simulink model "dbl_pendulum_total"  (R2021b)
settings: Solver=VariableStepAuto  StartTime=0.0  StopTime=10.0  RelTol=1e-3
values from neighbouring files (symbols this model uses):
  h = 0.001    [PID.m]    (also in blackbox_inpsig.m = fugiboard('Open', 'pendulum1'); blackbox_test.m = fugiboard('Open', 'pendulum1'); dbl_pend_blackbox_v1.m = fugiboard('Open', 'pendulum1'); dbl_pend_param_id_final.m)
libraries: eeLuenbergerObserver x1
settings Model: Creator=MICHAEL-LT  LastModifiedBy=mfuser
settings DataIOCC: ReturnWorkspaceOutputs=off

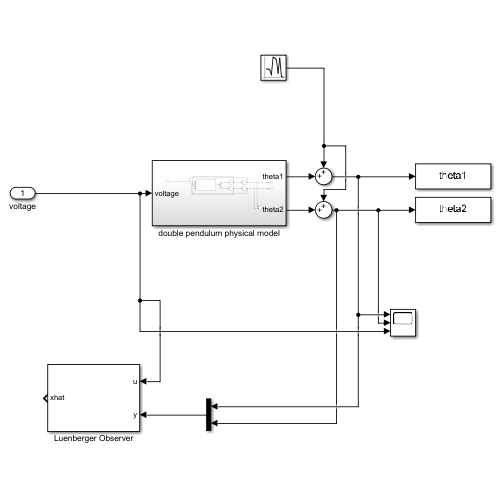
[thumbnail: Simulink's stored preview of the top-level diagram]
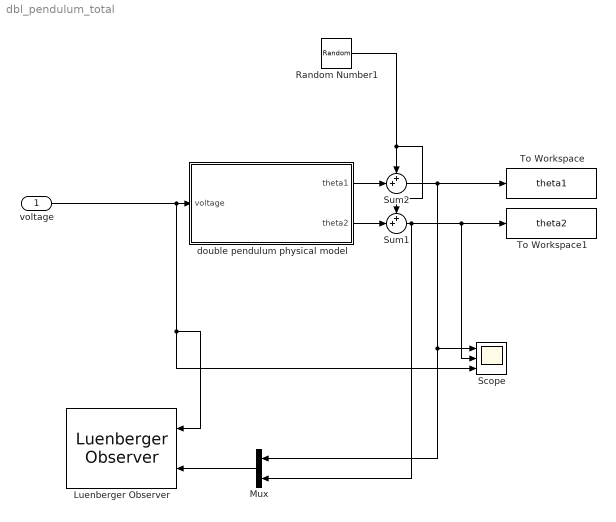
== system dbl_pendulum_total ==
  voltage : Inport
  Luenberger Observer : eeLuenbergerObserver/Luenberger Observer  StateSpaceType=Discrete-time  Ad=A_discr  Bd=B_discr  Cd=C_discr  Dd=D_discr  A=1  B=1  C=1  D=1  ObserverDesign=Observer gain  Ld=1  DesiredEigenvalues=0  x0=[0;0;0;0]  Tsd=0.1  Ts=h
      settings: SourceProductBaseCode=PS
  Mux : Mux  Inputs=2
  Random Number1 : RandomNumber  Variance=1e-5  SampleTime=h
  Scope : Scope  NumInputPorts=3
  Sum1 : Sum  Inputs=++|  SaturateOnIntegerOverflow=on
  Sum2 : Sum  Inputs=++|  SaturateOnIntegerOverflow=on
  To Workspace : ToWorkspace  VariableName=theta1  SampleTime=h
  To Workspace1 : ToWorkspace  VariableName=theta2  SampleTime=h
  double pendulum physical model : Subsystem
  wires:
  voltage/1 -> Scope/3, Luenberger Observer/1, double pendulum physical model/1(voltage)
  double pendulum physical model/1(theta1) -> Sum2/2
  Sum2/1 -> Mux/1, Scope/1, To Workspace/1
  double pendulum physical model/2(theta2) -> Sum1/2
  Sum1/1 -> Mux/2, Scope/2, To Workspace1/1
  Random Number1/1 -> Sum1/1, Sum2/1
  Mux/1 -> Luenberger Observer/2

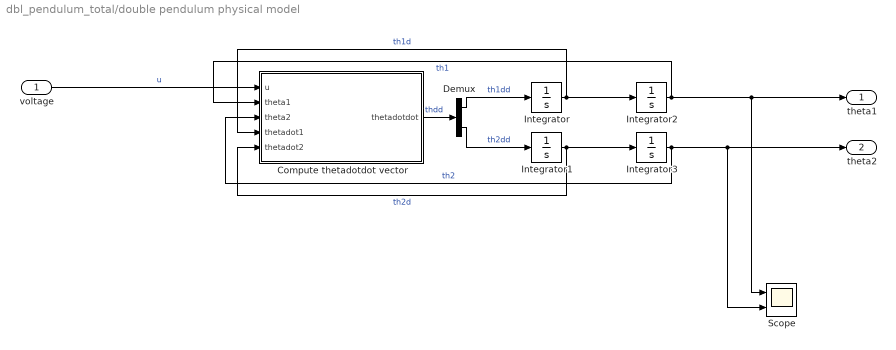
== system dbl_pendulum_total/double pendulum physical model ==
  voltage : Inport
  Compute thetadotdot vector : MATLAB Function  TreatAsAtomicUnit=on
  Demux : Demux  Outputs=2
  Integrator{,1..3} (4 alike) : Integrator
  Scope : Scope  NumInputPorts=2
  theta1 : Outport
  theta2 : Outport  Port=2
  wires:
  voltage/1 -> Compute thetadotdot vector/1(u)  "u"
  Compute thetadotdot vector/1(thetadotdot) -> Demux/1  "thdd"
  Demux/1 -> Integrator/1  "th1dd"
  Demux/2 -> Integrator1/1  "th2dd"
  Integrator/1 -> Compute thetadotdot vector/4(thetadot1), Integrator2/1  "th1d"
  Integrator1/1 -> Compute thetadotdot vector/5(thetadot2), Integrator3/1  "th2d"
  Integrator2/1 -> Compute thetadotdot vector/2(theta1), Scope/1, theta1/1  "th1"
  Integrator3/1 -> Compute thetadotdot vector/3(theta2), theta2/1, Scope/2  "th2"

== matlab function dbl_pendulum_total/double pendulum physical model/Compute thetadotdot vector ==
  data: u input; thetadotdot output; theta1 input; theta2 input; thetadot1 input; thetadot2 input
function thetadotdot  = get_thetadotdot(u, theta1, theta2, thetadot1, thetadot2)
%% Parameters (SI Units)
g = 9.81;
l1 = 0.1; % m, length of first link
l2 = 0.1; % m, length of second link
m1 = 0.125; % kg, mass of first link
m2 = 0.05;  % kg, mass of second link
c1 = -0.04; % m, center of mass of first link
c2 = 0.06;  % m, center of mass of second link
I1 = 0.074; % kg m^2, inertia of first link
I2 = 0.00012; % kg m^2, inertia of second link
b1 = 4.8;      % kg s^-1, damping of first joint
b2 = 0.0002;   % kg s^-1, damping of second joint
k_m = 50;      % Nm, motor gain
%tau_e = 0.03;  % s, motor electrical constant


%% Variables of the model
th1 = theta1;
th2 = theta2;
th1d = thetadot1;
th2d = thetadot2;
thd_vec = [th1d ; th2d];
thetadotdot = [0 ; 0];
T_vec = [k_m*u ; 0];

%% Matrices of physical model
P1 = m1 * c1 * c1 + m2 * l1 * l1 + I1;
P2 = m2 * c2 * c2 + I2;
P3 = m2 * l1 * c2;
g1 = (m1 * c1 + m2 * l1) * g;
g2 = m2 * c2 * g;

M = [[P1 + P2 + 2*P3*cos(th2), P2 + P3 * cos(th2)]; [P2 + P3 * cos(th2) P2]];
C = [[b1 - P3 * th2d * sin(th2), -P3 * (th1d + th2d)*sin(th2)]; [P3 * th1d * sin(th2), b2]];
G = [- g1 * sin(th1) - g2 * sin(th1 + th2); - g2 * sin(th1 + th2)];

%% Compute output angular acceleration
M_inv = inv(M);
thetadotdot = M_inv*T_vec - M_inv*C*thd_vec - M_inv*G;
